simulink model "modelo_atraso"  (R2021b)
settings: Solver=VariableStepAuto  StartTime=0.0  StopTime=600  RelTol=1e-3
model workspace (MAT data in the model file):
  Td = 2
  std_dev = 0.08
values from neighbouring files (symbols this model uses):
  C = pid(Kp, Ki, Kd)    [run_and_calculate.m]
  Ts = 0.1    [run_and_calculate.m]
libraries: cstblocks x11, slpidlib x4, commchan3 x1
settings Model: Creator=Gabriel Vieira  LastModifiedBy=Gabriel Vieira

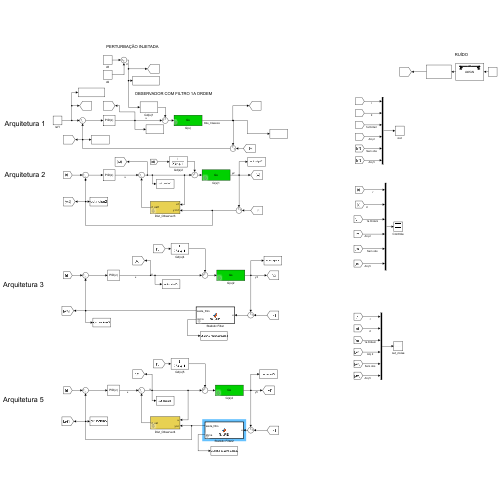
[thumbnail: Simulink's stored preview of the top-level diagram]
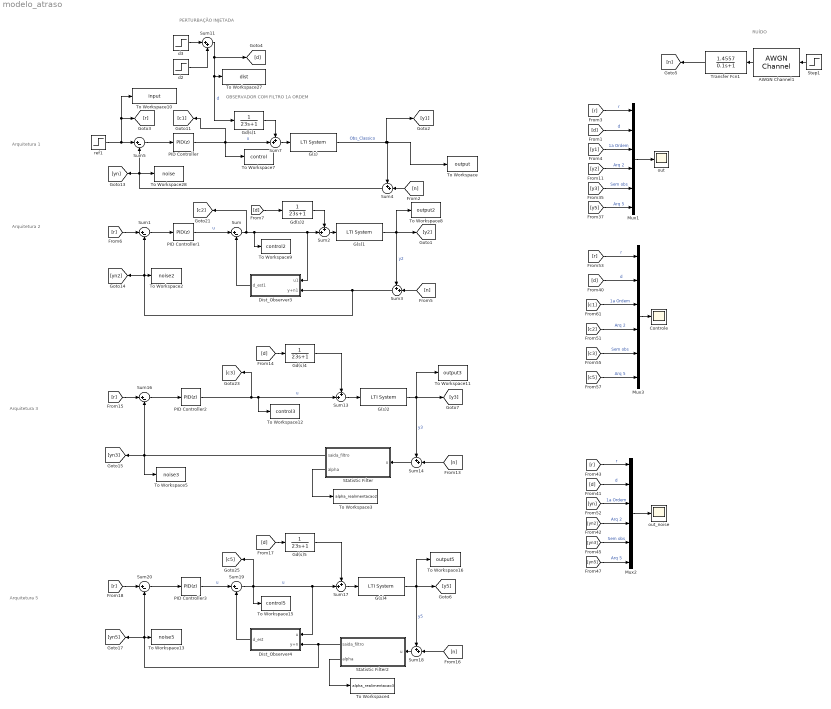
== system modelo_atraso ==
  note: OBSERVADOR COM FILTRO 1A ORDEM
  note: PERTURBAÇÃO INJETADA
  note: Arquitetura 1
  note: Arquitetura 2
  note: Arquitetura 3
  note: Arquitetura 5
  note: RUÍDO
  AWGN Channel1 : commchan3/AWGN Channel  InputProcessing=Columns as channels (frame based)  seed=67  noiseMode=Variance from mask  EbNodB=10  EsNodB=10  SNRdB=10  bitsPerSym=1  Ps=1  Tsym=1  variance=var_ruido
  Controle : Scope
  Dist_Observer3 : Subsystem  mask{Td=Td}
      mask prompts: Td "Filter time cte (Td)"
  Dist_Observer4 : Subsystem  mask{Td=Td}
      mask prompts: Td "Filter time cte (Td)"
  G(s){,1..2,4} (4 alike) : cstblocks/LTI System  sys=Gs  IC=[]
  Gd(s){1..2,4..5} (4 alike) : TransferFcn  Numerator=1  Denominator=[23 1]
  Mux1 : Mux  Inputs=6
  Mux2 : Mux  Inputs=6
  Mux3 : Mux  Inputs=6
  PID Controller{,1..3} (4 alike) : slpidlib/PID Controller  Controller=PID  Form=Parallel  TimeDomain=Discrete-time  UseExternalTs=off  SampleTime=-1  IntegratorMethod=Forward Euler  FilterMethod=Forward Euler  ControllerParametersSource=internal  P=C.Kp  I=C.Ki  D=C.Kd  UseFilter=off  N=100  TunerSelectOption=Transfer Function Based (PID Tuner App)  InitialConditionSource=internal  InitialConditionForIntegrator=0  InitialConditionForFilter=0  DifferentiatorICPrevScaledInput=0  ExternalReset=none  TrackingMode=off  Kt=1  LimitOutput=off  SatLimitsSource=internal  UpperSaturationLimit=inf  LowerSaturationLimit=-inf  LinearizeAsGain=on  AntiWindupMode=none  Kb=1  POutMin=[]  POutMax=[]  IOutMin=[]  IOutMax=[]  DOutMin=[]  DOutMax=[]  NOutMin=[]  NOutMax=[]  SumOutMin=[]  SumOutMax=[]  SaturationOutMin=[]  SaturationOutMax=[]  PParamMin=[]  PParamMax=[]  IParamMin=[]  IParamMax=[]  DParamMin=[]  DParamMax=[]  NParamMin=[]  NParamMax=[]  KbParamMin=[]  KbParamMax=[]  KtParamMin=[]  KtParamMax=[]  KbOutMin=[]  KbOutMax=[]  KtOutMin=[]  KtOutMax=[]  IntegratorOutMin=[]  IntegratorOutMax=[]  FilterOutMin=[]  FilterOutMax=[]  SumI1OutMin=[]  SumI1OutMax=[]  SumI2OutMin=[]  SumI2OutMax=[]  SumI3OutMin=[]  SumI3OutMax=[]  SumI4OutMin=[]  SumI4OutMax=[]  SumDOutMin=[]  SumDOutMax=[]  DifferentiatorOutMin=[]  DifferentiatorOutMax=[]  FilterDiffOutCoefMin=[]  FilterDiffOutCoefMax=[]  ReciprocalOutMin=[]  ReciprocalOutMax=[]  SumDenOutMin=[]  SumDenOutMax=[]  SumNumOutMin=[]  SumNumOutMax=[]  DivideOutMin=[]  DivideOutMax=[]  UdiffTsProdOutMin=[]  UdiffTsProdOutMax=[]  NTsProdOutMin=[]  NTsProdOutMax=[]  UintegralTsProdOutMin=[]  UintegralTsProdOutMax=[]  UngainTsProdOutMin=[]  UngainTsProdOutMax=[]  IntegratorContinuousStateAttributes=''  IntegratorStateMustResolveToSignalObject=off  IntegratorRTWStateStorageClass=Auto  FilterContinuousStateAttributes=''  FilterStateMustResolveToSignalObject=off  FilterRTWStateStorageClass=Auto  ParallelPVariant=InternalParameters  IdealPVariant=Disabled  IVariant=InternalParameters  DVariant=InternalParameters  IntegratorVariant=Discrete  SatVariant=Disabled  AWVariant=Passthrough  PCopyVariant=Disabled  TRVariant=Disabled  FdbkBlocksVariant=Forward  IdealPFdbkVariant=Disabled  SatFdbkVariant=Disabled  DerivativeFilterVariant=Differentiator  NVariant=Passthrough  NCopyVariant=Disabled_SignalSpec  FilterICVariant=InternalICsDifferentiator  IntegratorICVariant=InternalICs  ExternalResetVariant=Disabled  TRSumVariant=Passthrough  SumFdbkVariant=Disabled  SumVariant=Sum_PID  TsampFilterVariant=InternalTs  TsampNgainVariant=Passthrough  TsampIntegralVariant=Passthrough  ExternalSaturationOutDataTypeStr=Inherit: Same as second input
  Statistic Filter : MATLAB Function  TreatAsAtomicUnit=on  mask{std_dev=std_dev}
      mask prompts: std_dev "Noise Std Deviation (std_dev)"
  Statistic Filter2 : MATLAB Function  TreatAsAtomicUnit=on  mask{std_dev=std_dev/2}
      mask prompts: std_dev "Noise Std Deviation (std_dev)"
  Step1 : Step  Time=0  After=0  SampleTime=Ts
  Sum{,1,5,16,19..20} (6 alike) : Sum  Inputs=|+-
  Sum11 : Sum  Inputs=|++
  Sum{2..4,7,13..14,17..18} (8 alike) : Sum  Inputs=++|
  To Workspace : ToWorkspace  VariableName=output  SaveFormat=Timeseries  SampleTime=-1
  To Workspace10 : ToWorkspace  VariableName=input  SaveFormat=Timeseries  SampleTime=-1
  To Workspace11 : ToWorkspace  VariableName=output3  SaveFormat=Timeseries  SampleTime=-1
  To Workspace12 : ToWorkspace  VariableName=control3  SaveFormat=Timeseries  SampleTime=-1
  To Workspace13 : ToWorkspace  VariableName=noise5  SaveFormat=Timeseries  SampleTime=-1
  To Workspace15 : ToWorkspace  VariableName=control5  SaveFormat=Timeseries  SampleTime=-1
  To Workspace16 : ToWorkspace  VariableName=output5  SaveFormat=Timeseries  SampleTime=-1
  To Workspace2 : ToWorkspace  VariableName=noise2  SaveFormat=Timeseries  SampleTime=-1
  To Workspace27 : ToWorkspace  VariableName=dist  SaveFormat=Timeseries  SampleTime=-1
  To Workspace28 : ToWorkspace  VariableName=noise  SaveFormat=Timeseries  SampleTime=-1
  To Workspace3 : ToWorkspace  VariableName=alpha_realimentacao2  SaveFormat=Timeseries  SampleTime=-1
  To Workspace4 : ToWorkspace  VariableName=alpha_realimentacao3  SaveFormat=Timeseries  SampleTime=-1
  To Workspace5 : ToWorkspace  VariableName=noise3  SaveFormat=Timeseries  SampleTime=-1
  To Workspace7 : ToWorkspace  VariableName=control  SaveFormat=Timeseries  SampleTime=-1
  To Workspace8 : ToWorkspace  VariableName=output2  SaveFormat=Timeseries  SampleTime=-1
  To Workspace9 : ToWorkspace  VariableName=control2  SaveFormat=Timeseries  SampleTime=-1
  Transfer Fcn1 : TransferFcn  Numerator=[1.4557]  Denominator=[0.1 1]
  d2 : Step  Time=150  SampleTime=0
  d3 : Step  Time=200  After=-1  SampleTime=0
  out : Scope
  out_noise : Scope
  ref1 : Step  Time=50  SampleTime=0
  wires:
  Sum5/1 -> PID Controller/1
  d2/1 -> Sum11/2
  PID Controller/1 -> To Workspace7/1, Sum7/2, [c1]  "u"
  ref1/1 -> To Workspace10/1, [r], Sum5/1
  Mux1/1 -> out/1
  Sum7/1 -> G(s)/1
  Sum11/1 -> [d], To Workspace27/1, Gd(s)1/1  "d"
  [r] -> Mux1/1  "r"
  Gd(s)1/1 -> Sum7/1
  d3/1 -> Sum11/1
  [d] -> Mux1/2  "d"
  [n] -> Sum3/2
  Gd(s)2/1 -> Sum2/1
  Sum2/1 -> G(s)1/1
  Sum1/1 -> PID Controller1/1
  [r] -> Sum1/1
  [d] -> Gd(s)2/1
  PID Controller1/1 -> Sum/1  "u"
  Sum3/1 -> Dist_Observer3/2(y+n1), To Workspace2/1, [yn2], Sum1/2
  Dist_Observer3/1(d_est1) -> Sum/2
  G(s)1/1 -> [y2], To Workspace8/1, Sum3/1  "y2"
  [d] -> Gd(s)4/1
  Sum13/1 -> G(s)2/1
  Gd(s)4/1 -> Sum13/1
  [n] -> Sum14/2
  G(s)2/1 -> Sum14/1, To Workspace11/1, [y3]  "y3"
  Statistic Filter/2(alpha) -> To Workspace3/1
  Sum16/1 -> PID Controller2/1
  PID Controller2/1 -> [c3], To Workspace12/1, Sum13/2  "u"
  [r] -> Sum16/1
  Dist_Observer4/1(d_est) -> Sum19/2
  [r] -> Sum20/1
  Sum17/1 -> G(s)4/1
  Sum18/1 -> Statistic Filter2/1(u)
  Statistic Filter2/2(alpha) -> To Workspace4/1
  G(s)4/1 -> To Workspace16/1, [y5], Sum18/1  "y5"
  [d] -> Gd(s)5/1
  Sum20/1 -> PID Controller3/1
  PID Controller3/1 -> Sum19/1  "u"
  Gd(s)5/1 -> Sum17/1
  [n] -> Sum18/2
  [r] -> Mux2/1  "r"
  [d] -> Mux2/2  "d"
  Mux2/1 -> out_noise/1
  [yn] -> Mux2/3  "1a Ordem"
  Sum14/1 -> Statistic Filter/1(u)
  Statistic Filter2/1(saida_filtro) -> Dist_Observer4/2(y+n), To Workspace13/1, [yn5], Sum20/2
  [yn3] -> Mux2/5  "Sem obs"
  [yn2] -> Mux2/4  "Arq 2"
  [y2] -> Mux1/4  "Arq 2"
  [y3] -> Mux1/5  "Sem obs"
  Mux3/1 -> Controle/1
  Sum19/1 -> [c5], To Workspace15/1, Dist_Observer4/1(u), Sum17/2  "u"
  [c3] -> Mux3/5  "Sem obs"
  [r] -> Mux3/1  "r"
  [c1] -> Mux3/3  "1a Ordem"
  [d] -> Mux3/2  "d"
  [c2] -> Mux3/4  "Arq 2"
  Sum/1 -> [c2], To Workspace9/1, Dist_Observer3/1(u1), Sum2/2
  Statistic Filter/1(saida_filtro) -> To Workspace5/1, [yn3], Sum16/2
  [y5] -> Mux1/6  "Arq 5"
  [c5] -> Mux3/6  "Arq 5"
  [yn5] -> Mux2/6  "Arq 5"
  G(s)/1 -> [y1], To Workspace/1, Sum4/1  "Obs_Classico"
  Sum4/1 -> [yn], To Workspace28/1, Sum5/2
  Transfer Fcn1/1 -> [n]
  AWGN Channel1/1 -> Transfer Fcn1/1
  Step1/1 -> AWGN Channel1/1
  [n] -> Sum4/2
  [y1] -> Mux1/3  "1a Ordem"

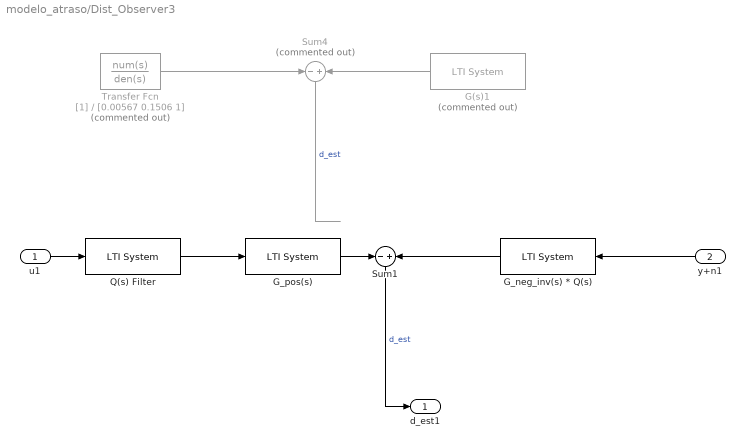
== system modelo_atraso/Dist_Observer3 ==
  u1 : Inport
  y+n1 : Inport  Port=2
  G(s)1 : cstblocks/LTI System  Commented=on  sys=G_neg_inv_Q  IC=[]
  G_neg_inv(s) * Q(s) : cstblocks/LTI System  sys=G_neg_inv_Q  IC=[]
  G_pos(s) : cstblocks/LTI System  sys=Gs_pos  IC=[]
  Q(s) Filter : cstblocks/LTI System  sys=Qs  IC=[]
  Sum1 : Sum  Inputs=-|+
  Sum4 : Sum  Commented=on  Inputs=-|+
  Transfer Fcn : TransferFcn  Commented=on  Denominator=[0.00567 0.1506 1]
  d_est1 : Outport
  wires:
  Transfer Fcn/1 -> Sum4/1
  Sum4/1 -> ?  "d_est"
  ? -> Transfer Fcn/1
  G(s)1/1 -> Sum4/2
  ? -> G(s)1/1
  G_pos(s)/1 -> Sum1/1
  y+n1/1 -> G_neg_inv(s) * Q(s)/1
  u1/1 -> Q(s) Filter/1
  Sum1/1 -> d_est1/1  "d_est"
  G_neg_inv(s) * Q(s)/1 -> Sum1/2
  Q(s) Filter/1 -> G_pos(s)/1

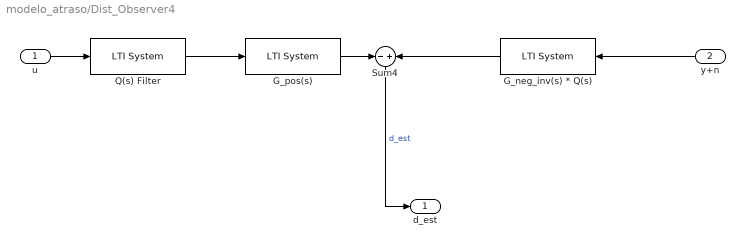
== system modelo_atraso/Dist_Observer4 ==
  u : Inport
  y+n : Inport  Port=2
  G_neg_inv(s) * Q(s) : cstblocks/LTI System  sys=G_neg_inv_Q  IC=[]
  G_pos(s) : cstblocks/LTI System  sys=Gs_pos  IC=[]
  Q(s) Filter : cstblocks/LTI System  sys=Qs  IC=[]
  Sum4 : Sum  Inputs=-|+
  d_est : Outport
  wires:
  Sum4/1 -> d_est/1  "d_est"
  u/1 -> Q(s) Filter/1
  G_neg_inv(s) * Q(s)/1 -> Sum4/2
  y+n/1 -> G_neg_inv(s) * Q(s)/1
  Q(s) Filter/1 -> G_pos(s)/1
  G_pos(s)/1 -> Sum4/1

== matlab function modelo_atraso/Statistic Filter2 ==
  settings: updateMethod=DISCRETE
  data: u input; saida_filtro output; std_dev parameter; alpha output
%Autor: Lucas Moura Gomes
%Filtro estatístico.

function [saida_filtro, alpha]  = filtroPID( u, std_dev)
    persistent x_ant;
    persistent alpha_orig;
    
    if isempty(x_ant)
        x_ant = 0;
        Ts = 0.01; %sampling time
        tf = 2; %continuous time cte.
        alpha_orig = 1 - exp(-1/tf * Ts); %c2d filter
    end
    
    alpha = erf(abs(x_ant - u)/(sqrt(2)*2*std_dev));
    
    if alpha > 1
        alpha = 1;
    end
    
    %up = 1.1; %upper bound 10%
    %alpha = alpha * alpha_orig * up;
    
    saida_filtro = (1-alpha)*x_ant + alpha*u;
    
    x_ant = saida_filtro;
end

%Autor: Lucas Moura Gomes
%Filtro estatístico.
% 
% function [saida_filtro, alpha] = filtroPID( u, erro_tipico_medicao, Tf  )
% 	
%     persistent x_ant;
%     
%     if isempty(x_ant)
%         x_ant = 0;
%     end
%     
%     Tf = Tf/1.5;
%     a_Tf = 1 - exp(-1/Tf * 5);
%     
%     alpha = erf(abs(x_ant - u)/(sqrt(2)*2*erro_tipico_medicao));
%     
%     if alpha > 1 
%         alpha = 1;
%     end;
%     
%     saida_filtro = (1-alpha)*x_ant + alpha*u;
% 
%     x_ant = saida_filtro;
%         
% 
%     saida_filtro = x_ant;
% 
%     
% end

== matlab function modelo_atraso/Statistic Filter ==
  settings: updateMethod=DISCRETE
  data: u input; saida_filtro output; std_dev parameter; alpha output
%Autor: Lucas Moura Gomes
%Filtro estatístico.

function [saida_filtro, alpha]  = filtroPID( u, std_dev)
    persistent x_ant;
    persistent alpha_orig;
    
    if isempty(x_ant)
        x_ant = 0;
        Ts = 0.01; %sampling time
        tf = 2; %continuous time cte.
        alpha_orig = 1 - exp(-1/tf * Ts); %c2d filter
    end
    
    alpha = erf(abs(x_ant - u)/(sqrt(2)*2*std_dev));
    
    if alpha > 1
        alpha = 1;
    end
    
    %up = 1.1; %upper bound 10%
    %alpha = alpha * alpha_orig * up;
    
    saida_filtro = (1-alpha)*x_ant + alpha*u;
    
    x_ant = saida_filtro;
end

%Autor: Lucas Moura Gomes
%Filtro estatístico.
% 
% function [saida_filtro, alpha] = filtroPID( u, erro_tipico_medicao, Tf  )
% 	
%     persistent x_ant;
%     
%     if isempty(x_ant)
%         x_ant = 0;
%     end
%     
%     Tf = Tf/1.5;
%     a_Tf = 1 - exp(-1/Tf * 5);
%     
%     alpha = erf(abs(x_ant - u)/(sqrt(2)*2*erro_tipico_medicao));
%     
%     if alpha > 1 
%         alpha = 1;
%     end;
%     
%     saida_filtro = (1-alpha)*x_ant + alpha*u;
% 
%     x_ant = saida_filtro;
%         
% 
%     saida_filtro = x_ant;
% 
%     
% end
